simulink model "Forward_current"  (R2015b)
settings: Solver=VariableStepAuto  StartTime=0.0  StopTime=1  RelTol=1e-6
values from neighbouring files (symbols this model uses):
  Kt = .07329    (= 0.07329)    [Parameters.m]
  N = 4    [Parameters.m]
undefined symbols (not defined in the file or in its folder): phi_r
libraries: fl_lib x6, pe_lib x3, nesl_utility x3
settings Model: Creator=Martin Andersen  LastModifiedBy=Martin Andersen

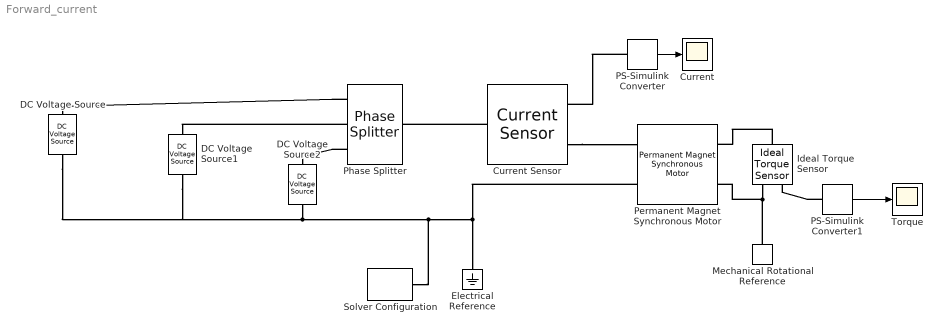
== system Forward_current ==
  Current : Scope
  Current Sensor : pe_lib/Sensors/Current Sensor
  DC Voltage Source : fl_lib/Electrical/Electrical Sources/DC Voltage Source  v0=Va V
  DC Voltage Source1 : fl_lib/Electrical/Electrical Sources/DC Voltage Source  v0=Vb V
  DC Voltage Source2 : fl_lib/Electrical/Electrical Sources/DC Voltage Source  v0=Vc V
  Electrical Reference : fl_lib/Electrical/Electrical Elements/Electrical Reference
  Ideal Torque Sensor : fl_lib/Mechanical/Mechanical Sensors/Ideal Torque Sensor
  Mechanical Rotational Reference : fl_lib/Mechanical/Rotational Elements/Mechanical Rotational Reference
  PS-Simulink Converter : nesl_utility/PS-Simulink Converter  PhysicalDomain=network_engine_domain  SubClassName=ps_output  LeftPortType=input  RightPortType=output  PseudoPeriodic=off  Frequencies=[]  Unit=1  AffineConversion=off
  PS-Simulink Converter1 : nesl_utility/PS-Simulink Converter  PhysicalDomain=network_engine_domain  SubClassName=ps_output  LeftPortType=input  RightPortType=output  PseudoPeriodic=off  Frequencies=[]  Unit=1  AffineConversion=off
  Permanent Magnet Synchronous Motor : pe_lib/Machines/Permanent Magnet Rotor/Permanent Magnet Synchronous Motor  nPolePairs=N  pm_flux_linkage=Kt/N Wb  stator_param=1  Ld=.1 mH  Lq=.1 mH  L0=.1 mH  Ls=0.0002 H  Lm=0.00002 H  Ms=0.00002 H  Rs=R Ohm  initial_currents=[0, 0, 0] A  axes_param=2  angular_position0=phi_r/N rad  rotor_offset=- pi / 2 rad  shift_3ph=[nan, nan, nan] rad  sqrt2OverSqrt3=nan  oneOverSqrt2=nan  twoPiOver3=nan  Lmin=1e-9 H
  Phase Splitter : pe_lib/Connections/Phase Splitter
  Solver Configuration : nesl_utility/Solver Configuration  PhysicalDomain=network_engine_domain  SubClassName=solver  LeftPortType=input  RightPortType=generic  Accelerate=off  Tones=[]  Harmonics=[]  SimulateNoise=off  Profile=off  UseLocalSampling=off  EnableSwitchedLinearOptims=on  FrequencyDomain=off  UseCCode=off  RelTol=0.001  AbsTol=1e-06  MinStep=1e-09  ToWorkspace=off  RevertToSquareIcSolve=off  NumHomotopyIterations=100  PhasorMode=off  PhasorModeNumHarmonics=1  DoDC=off  ResidualTolerance=1e-09  UseLocalSolver=off  LocalSolverChoice=NE_BACKWARD_EULER_ADVANCER  LocalSolverSampleTime=0.001  DoFixedCost=off  MaxNonlinIter=3  MaxModeIter=2  LinearAlgebra=Sparse  DelaysMemoryBudget=1024  AutomaticFiltering=on  FilteringTimeConstant=0.001
  Torque : Scope
  wires:
  PS-Simulink Converter1/1 -> Torque/1
  PS-Simulink Converter/1 -> Current/1
  connections:
  Permanent Magnet Synchronous Motor/LConn2 -- Electrical Reference/LConn1 -- Solver Configuration/RConn1 -- DC Voltage Source/RConn1 -- DC Voltage Source1/RConn1 -- DC Voltage Source2/RConn1
  Phase Splitter/RConn1 -- DC Voltage Source/LConn1
  Phase Splitter/RConn2 -- DC Voltage Source1/LConn1
  Phase Splitter/RConn3 -- DC Voltage Source2/LConn1
  Current Sensor/RConn2 -- Permanent Magnet Synchronous Motor/LConn1
  Current Sensor/LConn1 -- Phase Splitter/LConn1
  PS-Simulink Converter/LConn1 -- Current Sensor/RConn1
  Ideal Torque Sensor/RConn1 -- Permanent Magnet Synchronous Motor/RConn2 -- Mechanical Rotational Reference/LConn1
  Ideal Torque Sensor/LConn1 -- Permanent Magnet Synchronous Motor/RConn1
  PS-Simulink Converter1/LConn1 -- Ideal Torque Sensor/RConn2
